simulink model "animation"  (R2018b)
settings: Solver=VariableStepAuto  StartTime=0.0  StopTime=281.0754  FixedStep=0.01  RelTol=1e-3  EnableMultiTasking=on
values from neighbouring files (symbols this model uses):
  cm = [[0.3;49.6;82],[355.2;24;0.7],[9.8;0;36.7],[0.1;246;20],[0;13.9;55],[0;0;59]]    [dynamics.m]    (also in invDynController.m)
  D = generalizedInertiaMatrix(q,rho,DH,m,cm,I)    [dynamics.m]    (also in generalizedInertiaMatrix.m = D + (Si*J(:,:,i))'*Mc_i*(Si*J(:,:,i)); invDynController.m; motionPlanning.m = size(q_new,2); trajGen.m = size(q,1))
  m = [9 4.3 1.9 1.7 0.3 0.1]    [dynamics.m]    (also in invDynController.m)
  N = numel(pos_list)    [missionPlanning.m]    (also in motionPlanning.m = size(q_new,1); simManipulator.m = numel(Path(:,1)); trajGen.m = size(q,2); trajGen_fmincon.m = size(q,2))
undefined symbols (not defined in the file or in its folder): X, Y, Z
libraries: sm_lib x142, nesl_utility x51, simulink x2
(part 1 of 4)
settings Model: Creator=USER  LastModifiedBy=rabay
settings OptimizationCC: LifeSpan=inf
settings SFSimCC: SimUseLocalCustomCode=off
settings RTWCC: RTWUseLocalCustomCode=off
settings CodeAppCC: StateflowObjectComments=on
settings SimscapeCC: SimscapeNormalizeSystem=off

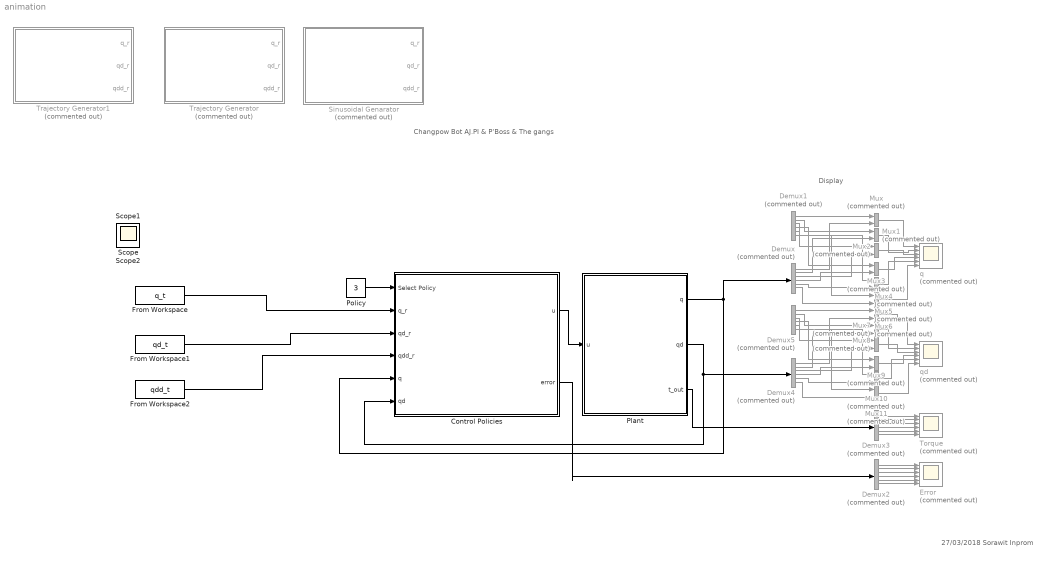
== system animation ==
  note: Display
  note: 27/03/2018
      | Sorawit Inprom
  note: Changpow Bot
      | AJ.PI & P'Boss & The gangs
  Control Policies : Subsystem  mask{Kp1=diag([10 10 10 10 10 10]), Kd1=diag([10 10 10 10 10 10]), Kp2=diag([10 10 10 10 10 10]), Kd2=diag([10 10 10 10 10 10]), max1=50, max2=30, max3=20, max4=20, max5=20, max6=20}
      mask prompts: Kp1 "Propotional Gain1"; Kd1 "Derivative Gain1"; Kp2 "Propotional Gain2"; Kd2 "Derivative Gain2"; max1 "Maximum Torque Joint1"; max2 "Maximum Torque Joint2"; max3 "Maximum Torque Joint3"; max4 "Maximum Torque Joint4"; max5 "Maximum Torque Joint5"; max6 "Maximum Torque Joint6"
      mask Display: image('C:\Users\dell\Downloads\29693766_2047918065235944_898913540_o.jpg');
  Demux{,1..5} (6 alike) : Demux  Commented=on  Outputs=6
  Error : Scope  Commented=on  NumInputPorts=6
  From Workspace : FromWorkspace  VariableName=q_t  SampleTime=0  Interpolate=off  OutputAfterFinalValue=Holding final value
  From Workspace1 : FromWorkspace  VariableName=qd_t  SampleTime=0  Interpolate=off  OutputAfterFinalValue=Holding final value
  From Workspace2 : FromWorkspace  VariableName=qdd_t  SampleTime=0  Interpolate=off  OutputAfterFinalValue=Holding final value
  Mux{,1..11} (12 alike) : Mux  Commented=on  Inputs=2
  Plant : Subsystem
  Policy : Constant  Value=3
  Sinusoidal Genarator : Subsystem  Commented=on  mask{a1=1, w1=pi*0.5}
      mask prompts: a1 "alpha"; w1 "omega"
  Torque : Scope  Commented=on  NumInputPorts=6
  Trajectory Generator : Subsystem  Commented=on  mask{T=10, q1=[2.504;0.367;0.569;-1.721;-0.122;1.7577], q2=[1.9908;-0.176;1.061;2;0.151;1.1145]}
      mask prompts: T "Time travel"; q1 "Goal Configuration Space1"; q2 "Goal Configuration Space2"
  Trajectory Generator1 : Subsystem  Commented=on  mask{T=5, q1=1, q2=0.5, q3=0.2, q4=0, q5=0, q6=0}
      mask prompts: T "Time travel"; q1 "Goal1"; q2 "Goal2"; q3 "Goal3"; q4 "Goal4"; q5 "Goal5"; q6 "Goal6"
  q : Scope  Commented=on  NumInputPorts=6
  qd : Scope  Commented=on  NumInputPorts=6
  Scope : Scope
  Scope1 : Scope
  Scope2 : Scope
  wires:
  Control Policies/1(u) -> Plant/1(u)
  Policy/1 -> Control Policies/1(Select Policy)
  Demux2/1 -> Error/1
  Demux1/5 -> Mux4/1
  Demux1/4 -> Mux3/1
  Demux3/1 -> Torque/1
  Demux3/2 -> Torque/2
  Demux3/3 -> Torque/3
  Demux/4 -> Mux3/2
  Demux/6 -> Mux5/2
  Demux1/3 -> Mux2/1
  Demux/3 -> Mux2/2
  Demux1/6 -> Mux5/1
  Demux1/2 -> Mux1/1
  Demux/1 -> Mux/2
  Control Policies/2(error) -> Demux2/1
  Demux/2 -> Mux1/2
  Mux2/1 -> q/3
  Demux/5 -> Mux4/2
  Demux5/1 -> Mux6/1
  Demux4/1 -> Mux6/2
  Mux6/1 -> qd/1
  Demux4/2 -> Mux7/2
  Demux4/3 -> Mux8/2
  Mux11/1 -> qd/6
  Mux8/1 -> qd/3
  Demux5/2 -> Mux7/1
  Mux7/1 -> qd/2
  Demux5/3 -> Mux8/1
  Mux9/1 -> qd/4
  Demux5/4 -> Mux9/1
  Demux4/4 -> Mux9/2
  Demux4/5 -> Mux10/2
  Demux5/6 -> Mux11/1
  Demux4/6 -> Mux11/2
  Demux5/5 -> Mux10/1
  Demux2/3 -> Error/3
  Demux1/1 -> Mux/1
  Demux2/2 -> Error/2
  Plant/1(q) -> Demux/1, Control Policies/5(q)
  Mux/1 -> q/1
  Plant/3(t_out) -> Demux3/1
  Mux1/1 -> q/2
  Plant/2(qd) -> Control Policies/6(qd), Demux4/1
  Mux3/1 -> q/4
  Mux4/1 -> q/5
  Mux5/1 -> q/6
  Mux10/1 -> qd/5
  Demux2/4 -> Error/4
  Demux2/5 -> Error/5
  Demux2/6 -> Error/6
  Demux3/4 -> Torque/4
  Demux3/5 -> Torque/5
  Demux3/6 -> Torque/6
  From Workspace/1 -> Control Policies/2(q_r)
  From Workspace1/1 -> Control Policies/3(qd_r)
  From Workspace2/1 -> Control Policies/4(qdd_r)

== system animation/Control Policies ==
  Select Policy : Inport
  q_r : Inport  Port=2
  qd_r : Inport  Port=3
  qdd_r : Inport  Port=4
  q : Inport  Port=5
  qd : Inport  Port=6
  Inverse Dynamics Control : Subsystem
  Mechanical Saturation : Subsystem
  Multiport Switch : MultiPortSwitch  DiagnosticForDefault=None
  PD Control : Subsystem
  PD Control with Gravity Compensator : Subsystem
  Sum : Sum  Inputs=|+-
  u : Outport
  error : Outport  Port=2
  wires:
  qd_r/1 -> PD Control/2(qd_r), Inverse Dynamics Control/2(qd_r), PD Control with Gravity Compensator/2(qd_r)
  q_r/1 -> PD Control/1(q_r), Sum/1, Inverse Dynamics Control/1(q_r), PD Control with Gravity Compensator/1(q_r)
  qdd_r/1 -> PD Control/3(qdd_r), Inverse Dynamics Control/3(qdd_r), PD Control with Gravity Compensator/3(qdd_r)
  q/1 -> PD Control/4(q), Sum/2, Inverse Dynamics Control/4(q), PD Control with Gravity Compensator/4("q ")
  qd/1 -> PD Control/5(qd), Inverse Dynamics Control/5(qd), PD Control with Gravity Compensator/5(qd)
  Select Policy/1 -> Multiport Switch/1
  Multiport Switch/1 -> Mechanical Saturation/1(t)
  Mechanical Saturation/1(t_sat) -> u/1
  Sum/1 -> error/1
  PD Control/1(u) -> Multiport Switch/2
  PD Control with Gravity Compensator/1(u) -> Multiport Switch/3
  Inverse Dynamics Control/1(u) -> Multiport Switch/4

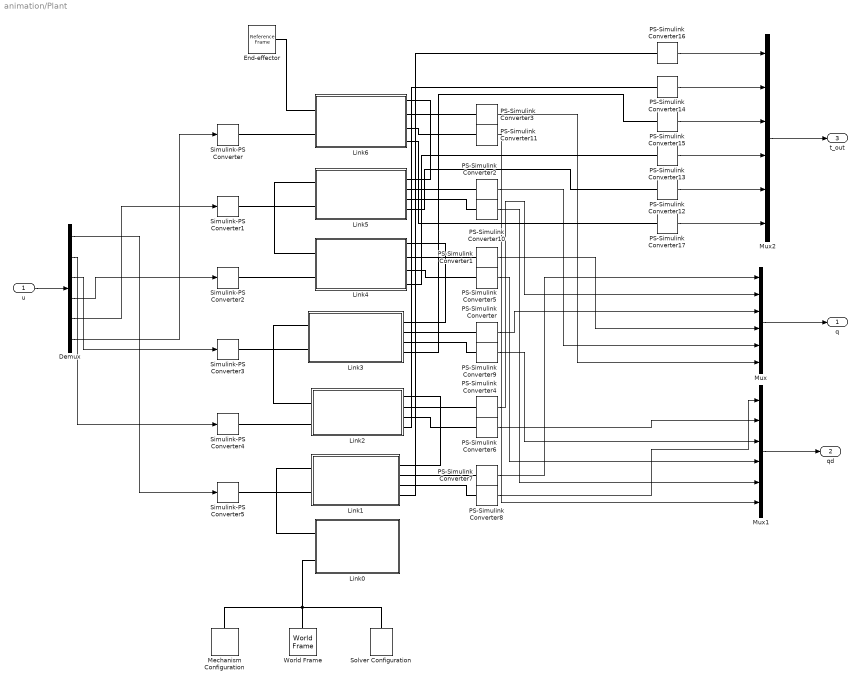
== system animation/Plant ==
  u : Inport
  Demux : Demux  Outputs=6
  End-effector : sm_lib/Frames and Transforms/Reference Frame
  Link0 : Subsystem
  Link1 : Subsystem
  Link2 : Subsystem
  Link3 : Subsystem
  Link4 : Subsystem
  Link5 : Subsystem
  Link6 : Subsystem
  Mechanism Configuration : sm_lib/Utilities/Mechanism Configuration  UniformGravity=Constant  GravityVector=[0 0 -9.80665]  GravityUnits=m/s^2  LinearizationDelta=0.001
  Mux : Mux  Inputs=6
  Mux1 : Mux  Inputs=6
  Mux2 : Mux  Inputs=6
  PS-Simulink Converter{,1..17} (18 alike) : nesl_utility/PS-Simulink Converter  PhysicalDomain=network_engine_domain  SubClassName=ps_output  LeftPortType=input  RightPortType=output  PseudoPeriodic=off  Frequencies=[]  Unit=1  AffineConversion=off
  Simulink-PS Converter{,1..5} (6 alike) : nesl_utility/Simulink-PS Converter  PhysicalDomain=network_engine_domain  SubClassName=ps_input  LeftPortType=input  RightPortType=output  PseudoPeriodic=off  Frequencies=[]  NoiseDistribution=none  NoiseParameters=[]  Unit=1  AffineConversion=off  FilteringAndDerivatives=zero  SimscapeFilterOrder=1  InputFilterTimeConstant=0.001  UdotUserProvided=1
  Solver Configuration : nesl_utility/Solver Configuration  PhysicalDomain=network_engine_domain  SubClassName=solver  LeftPortType=input  RightPortType=generic  Tones=[]  Harmonics=[]  SimulateNoise=off  Profile=off  UseLocalSampling=off  EnableSwitchedLinearOptims=on  FrequencyDomain=off  UseCCode=off  RelTol=0.001  AbsTol=1e-06  MinStep=1e-09  ToWorkspace=off  RevertToSquareIcSolve=off  NumHomotopyIterations=100  PhasorMode=off  PhasorModeNumHarmonics=1  DoDC=off  ResidualTolerance=1e-09  UseLocalSolver=off  LocalSolverChoice=NE_BACKWARD_EULER_ADVANCER  LocalSolverSampleTime=0.001  DoFixedCost=off  MaxNonlinIter=3  MaxModeIter=2  LinearAlgebra=Sparse  EquationFormulation=NE_TIME_EF  DelaysMemoryBudget=1024  AutomaticFiltering=on  FilteringTimeConstant=0.001  PartitionStorageMethod=AS_NEEDED  PartitionMemoryBudget=1024
  World Frame : sm_lib/Frames and Transforms/World Frame
  q : Outport
  qd : Outport  Port=2
  t_out : Outport  Port=3
  wires:
  Mux/1 -> q/1
  u/1 -> Demux/1
  Mux1/1 -> qd/1
  Mux2/1 -> t_out/1
  PS-Simulink Converter17/1 -> Mux2/6
  PS-Simulink Converter14/1 -> Mux2/2
  PS-Simulink Converter16/1 -> Mux2/1
  PS-Simulink Converter15/1 -> Mux2/3
  PS-Simulink Converter13/1 -> Mux2/4
  PS-Simulink Converter12/1 -> Mux2/5
  Demux/1 -> Simulink-PS Converter5/1
  Demux/2 -> Simulink-PS Converter4/1
  Demux/3 -> Simulink-PS Converter3/1
  Demux/4 -> Simulink-PS Converter2/1
  Demux/5 -> Simulink-PS Converter1/1
  Demux/6 -> Simulink-PS Converter/1
  PS-Simulink Converter3/1 -> Mux/6
  PS-Simulink Converter2/1 -> Mux/5
  PS-Simulink Converter1/1 -> Mux/4
  PS-Simulink Converter/1 -> Mux/3
  PS-Simulink Converter4/1 -> Mux/2
  PS-Simulink Converter7/1 -> Mux/1
  PS-Simulink Converter11/1 -> Mux1/6
  PS-Simulink Converter8/1 -> Mux1/1
  PS-Simulink Converter6/1 -> Mux1/2
  PS-Simulink Converter9/1 -> Mux1/3
  PS-Simulink Converter5/1 -> Mux1/4
  PS-Simulink Converter10/1 -> Mux1/5
  connections:
  World Frame/RConn1 -- Solver Configuration/RConn1 -- Link0/LConn2 -- Mechanism Configuration/RConn1
  Link1/RConn2 -- PS-Simulink Converter7/LConn1
  Link6/RConn2 -- PS-Simulink Converter3/LConn1
  Link3/RConn2 -- PS-Simulink Converter/LConn1
  Link2/RConn2 -- PS-Simulink Converter4/LConn1
  Simulink-PS Converter5/RConn1 -- Link1/LConn2
  Simulink-PS Converter4/RConn1 -- Link2/LConn2
  Link2/RConn1 -- Link1/RConn1
  Link1/LConn1 -- Link0/LConn1
  Simulink-PS Converter/RConn1 -- Link6/LConn2
  Simulink-PS Converter3/RConn1 -- Link3/LConn2
  Simulink-PS Converter2/RConn1 -- Link4/LConn2
  Simulink-PS Converter1/RConn1 -- Link5/LConn2
  Link4/RConn3 -- PS-Simulink Converter5/LConn1
  Link6/RConn3 -- PS-Simulink Converter11/LConn1
  Link5/RConn2 -- PS-Simulink Converter2/LConn1
  PS-Simulink Converter10/LConn1 -- Link5/RConn3
  PS-Simulink Converter8/LConn1 -- Link1/RConn3
  Link4/RConn1 -- Link3/RConn1
  Link5/LConn1 -- Link4/LConn1
  Link6/RConn1 -- Link5/RConn1
  Link3/LConn1 -- Link2/LConn1
  Link4/RConn2 -- PS-Simulink Converter1/LConn1
  PS-Simulink Converter9/LConn1 -- Link3/RConn3
  PS-Simulink Converter6/LConn1 -- Link2/RConn3
  End-effector/RConn1 -- Link6/LConn1
  Link6/RConn4 -- PS-Simulink Converter17/LConn1
  Link5/RConn4 -- PS-Simulink Converter12/LConn1
  Link4/RConn4 -- PS-Simulink Converter13/LConn1
  Link3/RConn4 -- PS-Simulink Converter15/LConn1
  Link2/RConn4 -- PS-Simulink Converter14/LConn1
  Link1/RConn4 -- PS-Simulink Converter16/LConn1

== system animation/Sinusoidal Genarator ==
  Clock : Clock
  Mux : Mux  Inputs=6
  Mux1 : Mux  Inputs=6
  Mux2 : Mux  Inputs=6
  Sin : Trigonometry
  Sin1 : Trigonometry  Operator=cos
  a1 : Gain  Gain=a1
  w1 : Gain  Gain=w1
  w3 : Gain  Gain=a1*w1
  w6 : Gain  Gain=-a1*w1^2
  q_r : Outport
  qd_r : Outport  Port=2
  qdd_r : Outport  Port=3
  wires:
  w3/1 -> Mux1/6, Mux1/5, Mux1/4, Mux1/3, Mux1/2, Mux1/1  "a1w1cos(w1t)"
  Sin/1 -> w6/1, a1/1
  w1/1 -> Sin1/1, Sin/1
  Clock/1 -> w1/1
  Mux/1 -> q_r/1
  Sin1/1 -> w3/1
  Mux1/1 -> qd_r/1
  Mux2/1 -> qdd_r/1
  w6/1 -> Mux2/6, Mux2/5, Mux2/4, Mux2/3, Mux2/2, Mux2/1  "-a1w1^2sin(w1t)"
  a1/1 -> Mux/6, Mux/5, Mux/4, Mux/3, Mux/2, Mux/1  "a1sin(w1t)"

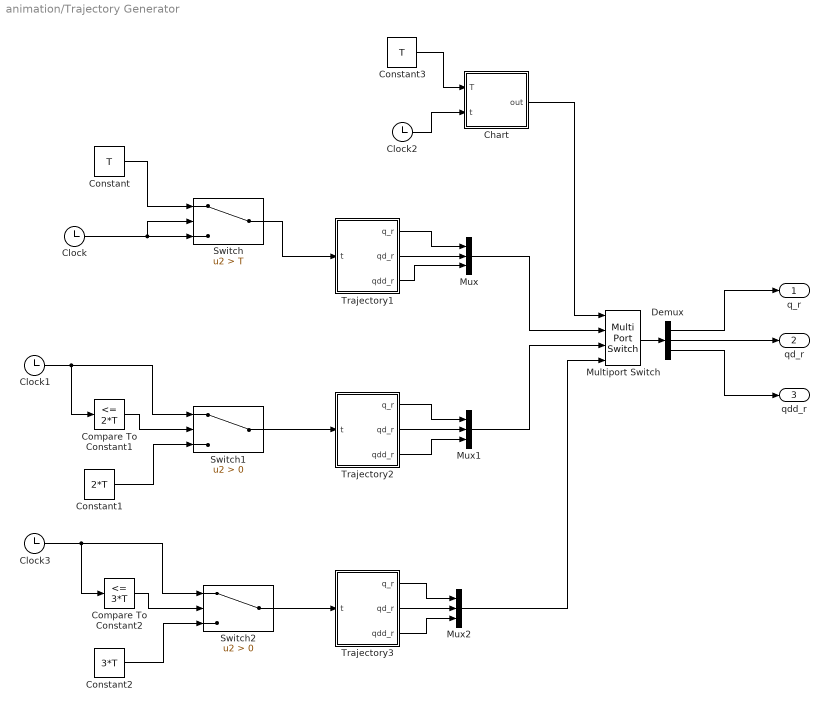
== system animation/Trajectory Generator ==
  Chart : Stateflow chart  TreatAsAtomicUnit=on
  Clock{,1..3} (4 alike) : Clock
  Compare To Constant1 : simulink/Logic and Bit Operations/Compare To Constant  relop=<=  const=2*T  OutDataTypeStr=uint8
  Compare To Constant2 : simulink/Logic and Bit Operations/Compare To Constant  relop=<=  const=3*T  OutDataTypeStr=uint8
  Constant : Constant  Value=T
  Constant1 : Constant  Value=2*T
  Constant2 : Constant  Value=3*T
  Constant3 : Constant  Value=T
  Demux : Demux  Outputs=3
  Multiport Switch : MultiPortSwitch  DiagnosticForDefault=None
  Mux : Mux  Inputs=3
  Mux1 : Mux  Inputs=3
  Mux2 : Mux  Inputs=3
  Switch : Switch  Criteria=u2 > Threshold  Threshold=T
  Switch1 : Switch  Criteria=u2 > Threshold
  Switch2 : Switch  Criteria=u2 > Threshold
  Trajectory1 : Subsystem
  Trajectory2 : Subsystem
  Trajectory3 : Subsystem
  q_r : Outport
  qd_r : Outport  Port=2
  qdd_r : Outport  Port=3
  wires:
  Clock/1 -> Switch/2, Switch/3
  Constant/1 -> Switch/1
  Switch/1 -> Trajectory1/1(t)
  Switch1/1 -> Trajectory2/1(t)
  Trajectory1/1(q_r) -> Mux/1
  Trajectory1/2(qd_r) -> Mux/2
  Trajectory1/3(qdd_r) -> Mux/3
  Trajectory2/2(qd_r) -> Mux1/2
  Trajectory2/1(q_r) -> Mux1/1
  Trajectory2/3(qdd_r) -> Mux1/3
  Mux/1 -> Multiport Switch/2
  Mux1/1 -> Multiport Switch/3
  Clock2/1 -> Chart/2(t)
  Multiport Switch/1 -> Demux/1
  Constant1/1 -> Switch1/3
  Clock1/1 -> Switch1/1, Compare To Constant1/1
  Compare To Constant1/1 -> Switch1/2
  Compare To Constant2/1 -> Switch2/2
  Clock3/1 -> Compare To Constant2/1, Switch2/1
  Constant2/1 -> Switch2/3
  Switch2/1 -> Trajectory3/1(t)
  Trajectory3/2(qd_r) -> Mux2/2
  Trajectory3/1(q_r) -> Mux2/1
  Trajectory3/3(qdd_r) -> Mux2/3
  Mux2/1 -> Multiport Switch/4
  Constant3/1 -> Chart/1(T)
  Chart/1(out) -> Multiport Switch/1
  Demux/1 -> q_r/1
  Demux/2 -> qd_r/1
  Demux/3 -> qdd_r/1

== system animation/Trajectory Generator1 ==
  Clock1 : Clock
  Constant1 : Constant  Value=T
  Switch1 : Switch  Criteria=u2 > Threshold  Threshold=T
  Trajectory2 : Subsystem
  q_r : Outport
  qd_r : Outport  Port=2
  qdd_r : Outport  Port=3
  wires:
  Trajectory2/3(qdd_r) -> qdd_r/1
  Constant1/1 -> Switch1/1
  Trajectory2/1(q_r) -> q_r/1
  Clock1/1 -> Switch1/2, Switch1/3
  Trajectory2/2(qd_r) -> qd_r/1
  Switch1/1 -> Trajectory2/1(t)

== system animation/Control Policies/Inverse Dynamics Control ==
  q_r : Inport
  qd_r : Inport  Port=2
  qdd_r : Inport  Port=3
  q : Inport  Port=4
  qd : Inport  Port=5
  Inverse Dynamics : Subsystem
  Outer_loop : Subsystem
  u : Outport
  wires:
  qd_r/1 -> Outer_loop/2(qd_r)
  q/1 -> Inverse Dynamics/2(q), Outer_loop/4(q)
  qd/1 -> Inverse Dynamics/3(qd), Outer_loop/5(qd)
  Outer_loop/1(a) -> Inverse Dynamics/1(a)
  qdd_r/1 -> Outer_loop/3(qdd_r)
  q_r/1 -> Outer_loop/1(q_r)
  Inverse Dynamics/1("Torque ") -> u/1

== system animation/Control Policies/Mechanical Saturation ==
  t : Inport
  Demux3 : Demux  Outputs=6
  Mux : Mux  Inputs=6
  Saturation : Saturate  UpperLimit=max1  LowerLimit=-max1
  Saturation1 : Saturate  UpperLimit=max2  LowerLimit=-max2
  Saturation2 : Saturate  UpperLimit=max3  LowerLimit=-max3
  Saturation3 : Saturate  UpperLimit=max4  LowerLimit=-max4
  Saturation4 : Saturate  UpperLimit=max5  LowerLimit=-max5
  Saturation5 : Saturate  UpperLimit=max6  LowerLimit=-max6
  t_sat : Outport
  wires:
  Demux3/3 -> Saturation2/1
  Saturation2/1 -> Mux/3
  t/1 -> Demux3/1
  Demux3/4 -> Saturation3/1
  Saturation3/1 -> Mux/4
  Demux3/2 -> Saturation1/1
  Saturation/1 -> Mux/1
  Saturation1/1 -> Mux/2
  Demux3/6 -> Saturation5/1
  Saturation5/1 -> Mux/6
  Demux3/5 -> Saturation4/1
  Mux/1 -> t_sat/1
  Saturation4/1 -> Mux/5
  Demux3/1 -> Saturation/1

== system animation/Control Policies/PD Control ==
  q_r : Inport
  qd_r : Inport  Port=2
  qdd_r : Inport  Port=3
  q : Inport  Port=4
  qd : Inport  Port=5
  Kd3 : Gain  Gain=Kd2  Multiplication=Matrix(K*u)
  Kp3 : Gain  Gain=Kp2  Multiplication=Matrix(K*u)
  Sum12 : Sum  Inputs=|+-
  Sum13 : Sum  Inputs=|++
  Sum8 : Sum  Inputs=|+-
  u : Outport
  wires:
  q_r/1 -> Sum8/1
  qd/1 -> Sum12/2
  Kd3/1 -> Sum13/2
  qd_r/1 -> Sum12/1
  Sum12/1 -> Kd3/1  "eqd"
  q/1 -> Sum8/2
  Kp3/1 -> Sum13/1
  Sum8/1 -> Kp3/1  "eq"
  Sum13/1 -> u/1

== system animation/Control Policies/PD Control with Gravity Compensator ==
  q_r : Inport
  qd_r : Inport  Port=2
  qdd_r : Inport  Port=3
  "q " : Inport  Port=4
  qd : Inport  Port=5
  Gravity Compensator : Subsystem
  PD control : Subsystem
  u : Outport
  wires:
  PD control/1(u) -> u/1
  Gravity Compensator/1("Torque ") -> PD control/1(compensate)
  q_r/1 -> PD control/2(q_r)
  qd/1 -> PD control/5(qd)
  qd_r/1 -> PD control/3(qd_r)
  "q "/1 -> PD control/4(q), Gravity Compensator/1(q)

== system animation/Plant/Link0 ==
  Rigid Transform : sm_lib/Frames and Transforms/Rigid Transform  TranslationMethod=None  TranslationStandardOffset=0  TranslationLengthUnit=m  TranslationStandardAxis=+Z  TranslationCartesianOffset=[0 0 0]  TranslationROffset=0  TranslationROffsetUnits=m  TranslationZOffset=0  TranslationZOffsetUnits=m  TranslationThetaOffset=0  TranslationThetaOffsetUnits=deg  RotationMethod=StandardAxis  RotationAngleUnits=rad  RotationStandardAxis=+Z  RotationAngle=pi  RotationArbitraryAxis=[0 0 1]  FollAlignAxisA=+X  BaseAlignAxisA=+Y  FollAlignAxisB=+Y  BaseAlignAxisB=+Z  RotationSequenceAxes=FollowerAxes  RotationSequence=XYX  RotationSequenceAngles=[0 0 0]  RotationSequenceAnglesUnits=deg  RotationMatrix=[1 0 0; 0 1 0; 0 0 1]
  Solid : sm_lib/Body Elements/Solid  InertiaType=Custom  Mass=12.21  MassUnits=kg  CenterOfMass=[53.3 2.09 37.75]  CenterOfMassUnits=mm  MomentsOfInertia=[0.27 0.33 0.54]  MomentsOfInertiaUnits=kg*m^2  ProductsOfInertia=[0 0.03 0.01]  ProductsOfInertiaUnits=kg*m^2  BasedOnType=Density  Density=1000  DensityUnits=kg/m^3  DoExposeReferenceFrame=on  SerializedFrames=<Frames/>  GraphicType=FromGeometry  MarkerShape=Sphere  MarkerSize=10  GraphicVisPropType=SimpleVisualProperties  GraphicDiffuseColor=[0.5 0.5 0.5]  GraphicSpecularColor=[0.5 0.5 0.5 1.0]  GraphicAmbientColor=[0.15 0.15 0.15 1.0]  GraphicEmissiveColor=[0.0 0.0 0.0 1.0]  GraphicShininess=75  GraphicOpacity=1.0  GeometryShape=FromFile  RectangleSize=[1 1]  RectangleSizeUnits=m  BrickDimensions=[1 1 1]  BrickDimensionUnits=m  CylinderRadius=1  CylinderRadiusUnits=m  CylinderLength=1  CylinderLengthUnits=m  SphereRadius=1  SphereRadiusUnits=m  EllipsoidRadii=[1 1 1]  EllipsoidRadiiUnits=m  ExtrusionCrossSection=[1 1; -1 1; -1 -1; 1 -1]  ExtrusionCrossSectionUnits=m  ExtrusionLength=1  ExtrusionLengthUnits=m  PolygonNumSides=3  PolygonOuterRadius=1  PolygonOuterRadiusUnits=m  ExtGeomFileType=STL  ExtGeomFileName=C:\Users\dell\Desktop\module8&9\Intro to robotics\Project\CAD\Assem0+frame.STL  ExtGeomFileUnits=mm  RevolutionCrossSection=[1 1; 1 -1; 2 -1; 2 1]  RevolutionCrossSectionUnits=m  RevolutionExtent=Full  RevolutionAngle=180  RevolutionAngleUnits=deg
  Solid1 : sm_lib/Body Elements/Solid  InertiaType=Custom  Mass=1  MassUnits=kg  CenterOfMass=[0 0 0]  CenterOfMassUnits=m  MomentsOfInertia=[1 1 1]  MomentsOfInertiaUnits=kg*m^2  ProductsOfInertia=[0 0 0]  ProductsOfInertiaUnits=kg*m^2  BasedOnType=Density  Density=1000  DensityUnits=kg/(m^3)  DoExposeReferenceFrame=on  SerializedFrames=<Frames/>  GraphicType=FromGeometry  MarkerShape=Sphere  MarkerSize=10  GraphicVisPropType=SimpleVisualProperties  GraphicDiffuseColor=[0.5 0.5 0.5]  GraphicSpecularColor=[0.5 0.5 0.5 1.0]  GraphicAmbientColor=[0.15 0.15 0.15 1.0]  GraphicEmissiveColor=[0.0 0.0 0.0 1.0]  GraphicShininess=75  GraphicOpacity=1.0  GeometryShape=FromFile  RectangleSize=[1 1]  RectangleSizeUnits=m  BrickDimensions=[1 1 1]  BrickDimensionUnits=m  CylinderRadius=1  CylinderRadiusUnits=m  CylinderLength=1  CylinderLengthUnits=m  SphereRadius=1  SphereRadiusUnits=m  EllipsoidRadii=[1 1 1]  EllipsoidRadiiUnits=m  ExtrusionCrossSection=[1 1; -1 1; -1 -1; 1 -1]  ExtrusionCrossSectionUnits=m  ExtrusionLength=1  ExtrusionLengthUnits=m  PolygonNumSides=3  PolygonOuterRadius=1  PolygonOuterRadiusUnits=m  ExtGeomFileType=STL  ExtGeomFileName=D:\Chin\3rdYearsProject\IntroRobotics\Project\CAD\Workspace_with_Plate.STL  ExtGeomFileUnits=mm  RevolutionCrossSection=[1 1; 1 -1; 2 -1; 2 1]  RevolutionCrossSectionUnits=m  RevolutionExtent=Full  RevolutionAngle=180  RevolutionAngleUnits=deg
  Frame0 : PMIOPort  Side=Left
  World Frame : PMIOPort  Port=2  Side=Left
  connections:
  Solid/RConn1 -- Solid1/RConn1 -- Rigid Transform/RConn1 -- Frame0/RConn1
  World Frame/RConn1 -- Rigid Transform/LConn1

== system animation/Plant/Link1 ==
  Reference Frame : sm_lib/Frames and Transforms/Reference Frame
  Revolute Joint : sm_lib/Joints/Revolute Joint  SenseConstraintForce=off  SenseConstraintForceX=off  SenseConstraintForceY=off  SenseConstraintForceZ=off  SenseConstraintTorque=off  SenseConstraintTorqueX=off  SenseConstraintTorqueY=off  SenseConstraintTorqueZ=off  SenseTotalForce=off  SenseTotalForceX=off  SenseTotalForceY=off  SenseTotalForceZ=off  SenseTotalTorque=off  SenseTotalTorqueX=off  SenseTotalTorqueY=off  SenseTotalTorqueZ=off  CompositeWrenchDir=FollowerOnBase  CompositeWrenchFrame=BaseFrame  EquilibriumPosition=0  EquilibriumPositionUnits=deg  SpringStiffness=0  SpringStiffnessUnits=N*m/deg  DampingCoefficient=0  DampingCoefficientUnits=N*m/(deg/s)  TorqueActuationMode=InputTorque  MotionActuationMode=ComputedMotion  SensePosition=on  SenseVelocity=on  SenseAcceleration=off  SenseTorqueForce=on  PositionTargetSpecify=on  PositionTargetPriority=High  PositionTargetValue=0  PositionTargetValueUnits=deg  VelocityTargetSpecify=on  VelocityTargetPriority=High  VelocityTargetValue=0  VelocityTargetValueUnits=deg/s
  Rigid Transform1 : sm_lib/Frames and Transforms/Rigid Transform  TranslationMethod=None  TranslationStandardOffset=0  TranslationLengthUnit=m  TranslationStandardAxis=+Z  TranslationCartesianOffset=[0 0 0]  TranslationROffset=0  TranslationROffsetUnits=m  TranslationZOffset=0  TranslationZOffsetUnits=m  TranslationThetaOffset=0  TranslationThetaOffsetUnits=deg  RotationMethod=StandardAxis  RotationAngleUnits=rad  RotationStandardAxis=+Z  RotationAngle=-pi/2  RotationArbitraryAxis=[0 0 1]  FollAlignAxisA=+X  BaseAlignAxisA=+Y  FollAlignAxisB=+Y  BaseAlignAxisB=+Z  RotationSequenceAxes=FollowerAxes  RotationSequence=XYX  RotationSequenceAngles=[0 0 0]  RotationSequenceAnglesUnits=deg  RotationMatrix=[1 0 0; 0 1 0; 0 0 1]
  Rigid Transform17 : sm_lib/Frames and Transforms/Rigid Transform  TranslationMethod=None  TranslationStandardOffset=500  TranslationLengthUnit=mm  TranslationStandardAxis=+X  TranslationCartesianOffset=[0 0 0]  TranslationROffset=0  TranslationROffsetUnits=m  TranslationZOffset=0  TranslationZOffsetUnits=m  TranslationThetaOffset=0  TranslationThetaOffsetUnits=deg  RotationMethod=StandardAxis  RotationAngleUnits=rad  RotationStandardAxis=+X  RotationAngle=pi/2  RotationArbitraryAxis=[0 0 1]  FollAlignAxisA=+X  BaseAlignAxisA=+Y  FollAlignAxisB=+Y  BaseAlignAxisB=+Z  RotationSequenceAxes=FollowerAxes  RotationSequence=XYX  RotationSequenceAngles=[0 0 0]  RotationSequenceAnglesUnits=deg  RotationMatrix=[1 0 0; 0 1 0; 0 0 1]
  Rigid Transform2 : sm_lib/Frames and Transforms/Rigid Transform  TranslationMethod=StandardAxis  TranslationStandardOffset=250.5  TranslationLengthUnit=mm  TranslationStandardAxis=+Z  TranslationCartesianOffset=[0 0 0]  TranslationROffset=0  TranslationROffsetUnits=m  TranslationZOffset=0  TranslationZOffsetUnits=m  TranslationThetaOffset=0  TranslationThetaOffsetUnits=deg  RotationMethod=None  RotationAngleUnits=deg  RotationStandardAxis=+Z  RotationAngle=0.0  RotationArbitraryAxis=[0 0 1]  FollAlignAxisA=+X  BaseAlignAxisA=+Y  FollAlignAxisB=+Y  BaseAlignAxisB=+Z  RotationSequenceAxes=FollowerAxes  RotationSequence=XYX  RotationSequenceAngles=[0 0 0]  RotationSequenceAnglesUnits=deg  RotationMatrix=[1 0 0; 0 1 0; 0 0 1]
  Rigid Transform3 : sm_lib/Frames and Transforms/Rigid Transform  TranslationMethod=None  TranslationStandardOffset=0  TranslationLengthUnit=m  TranslationStandardAxis=+Z  TranslationCartesianOffset=[0 0 0]  TranslationROffset=0  TranslationROffsetUnits=m  TranslationZOffset=0  TranslationZOffsetUnits=m  TranslationThetaOffset=0  TranslationThetaOffsetUnits=deg  RotationMethod=None  RotationAngleUnits=rad  RotationStandardAxis=+X  RotationAngle=pi/2  RotationArbitraryAxis=[0 0 1]  FollAlignAxisA=+X  BaseAlignAxisA=+Y  FollAlignAxisB=+Y  BaseAlignAxisB=+Z  RotationSequenceAxes=FollowerAxes  RotationSequence=XYX  RotationSequenceAngles=[0 0 0]  RotationSequenceAnglesUnits=deg  RotationMatrix=[1 0 0; 0 1 0; 0 0 1]
  Solid1 : sm_lib/Body Elements/Solid  InertiaType=Custom  Mass=8.44  MassUnits=kg  CenterOfMass=[0.26 -62.55 100.99]  CenterOfMassUnits=mm  MomentsOfInertia=[0.25 0.21 0.09]  MomentsOfInertiaUnits=kg*m^2  ProductsOfInertia=[-0.02 0 0]  ProductsOfInertiaUnits=kg*m^2  BasedOnType=Density  Density=1000  DensityUnits=kg/m^3  DoExposeReferenceFrame=on  SerializedFrames=<Frames/>  GraphicType=FromGeometry  MarkerShape=Sphere  MarkerSize=10  GraphicVisPropType=SimpleVisualProperties  GraphicDiffuseColor=[0.0 0.0 1.0]  GraphicSpecularColor=[0.5 0.5 0.5 1.0]  GraphicAmbientColor=[0.15 0.15 0.15 1.0]  GraphicEmissiveColor=[0.0 0.0 0.0 1.0]  GraphicShininess=75  GraphicOpacity=1.0  GeometryShape=FromFile  RectangleSize=[1 1]  RectangleSizeUnits=m  BrickDimensions=[1 1 1]  BrickDimensionUnits=m  CylinderRadius=1  CylinderRadiusUnits=m  CylinderLength=1  CylinderLengthUnits=m  SphereRadius=1  SphereRadiusUnits=m  EllipsoidRadii=[1 1 1]  EllipsoidRadiiUnits=m  ExtrusionCrossSection=[1 1; -1 1; -1 -1; 1 -1]  ExtrusionCrossSectionUnits=m  ExtrusionLength=1  ExtrusionLengthUnits=m  PolygonNumSides=3  PolygonOuterRadius=1  PolygonOuterRadiusUnits=m  ExtGeomFileType=STL  ExtGeomFileName=D:\Chin\3rdYearsProject\IntroRobotics\Project\CAD\Assem2+1.STL  ExtGeomFileUnits=mm  RevolutionCrossSection=[1 1; 1 -1; 2 -1; 2 1]  RevolutionCrossSectionUnits=m  RevolutionExtent=Full  RevolutionAngle=180  RevolutionAngleUnits=deg
  Frame1 : PMIOPort  Side=Right
  Frame0 : PMIOPort  Port=2  Side=Left
  q : PMIOPort  Port=3  Side=Right
  w : PMIOPort  Port=4  Side=Right
  t : PMIOPort  Port=5  Side=Left
  t_out : PMIOPort  Port=6  Side=Right
  connections:
  Rigid Transform17/RConn1 -- Frame1/RConn1 -- Solid1/RConn1 -- Reference Frame/RConn1
  Rigid Transform3/RConn1 -- Rigid Transform17/LConn1
  Rigid Transform3/LConn1 -- Rigid Transform2/RConn1
  Rigid Transform1/LConn1 -- Revolute Joint/RConn1
  Rigid Transform2/LConn1 -- Rigid Transform1/RConn1
  Revolute Joint/RConn2 -- q/RConn1
  Revolute Joint/LConn1 -- Frame0/RConn1
  Revolute Joint/RConn3 -- w/RConn1
  t/RConn1 -- Revolute Joint/LConn2
  Revolute Joint/RConn4 -- t_out/RConn1

== system animation/Plant/Link2 ==
  Reference Frame1 : sm_lib/Frames and Transforms/Reference Frame
  Revolute Joint1 : sm_lib/Joints/Revolute Joint  SenseConstraintForce=off  SenseConstraintForceX=off  SenseConstraintForceY=off  SenseConstraintForceZ=off  SenseConstraintTorque=off  SenseConstraintTorqueX=off  SenseConstraintTorqueY=off  SenseConstraintTorqueZ=off  SenseTotalForce=off  SenseTotalForceX=off  SenseTotalForceY=off  SenseTotalForceZ=off  SenseTotalTorque=off  SenseTotalTorqueX=off  SenseTotalTorqueY=off  SenseTotalTorqueZ=off  CompositeWrenchDir=FollowerOnBase  CompositeWrenchFrame=BaseFrame  EquilibriumPosition=0  EquilibriumPositionUnits=deg  SpringStiffness=0  SpringStiffnessUnits=N*m/deg  DampingCoefficient=0  DampingCoefficientUnits=N*m/(deg/s)  TorqueActuationMode=InputTorque  MotionActuationMode=ComputedMotion  SensePosition=on  SenseVelocity=on  SenseAcceleration=off  SenseTorqueForce=on  PositionTargetSpecify=on  PositionTargetPriority=High  PositionTargetValue=0  PositionTargetValueUnits=deg  VelocityTargetSpecify=on  VelocityTargetPriority=High  VelocityTargetValue=0  VelocityTargetValueUnits=deg/s
  Rigid Transform16 : sm_lib/Frames and Transforms/Rigid Transform  TranslationMethod=None  TranslationStandardOffset=500  TranslationLengthUnit=mm  TranslationStandardAxis=+X  TranslationCartesianOffset=[0 0 0]  TranslationROffset=0  TranslationROffsetUnits=m  TranslationZOffset=0  TranslationZOffsetUnits=m  TranslationThetaOffset=0  TranslationThetaOffsetUnits=deg  RotationMethod=None  RotationAngleUnits=deg  RotationStandardAxis=+Z  RotationAngle=0.0  RotationArbitraryAxis=[0 0 1]  FollAlignAxisA=+X  BaseAlignAxisA=+Y  FollAlignAxisB=+Y  BaseAlignAxisB=+Z  RotationSequenceAxes=FollowerAxes  RotationSequence=XYX  RotationSequenceAngles=[0 0 0]  RotationSequenceAnglesUnits=deg  RotationMatrix=[1 0 0; 0 1 0; 0 0 1]
  Rigid Transform4 : sm_lib/Frames and Transforms/Rigid Transform  TranslationMethod=None  TranslationStandardOffset=0  TranslationLengthUnit=m  TranslationStandardAxis=+Z  TranslationCartesianOffset=[0 0 0]  TranslationROffset=0  TranslationROffsetUnits=m  TranslationZOffset=0  TranslationZOffsetUnits=m  TranslationThetaOffset=0  TranslationThetaOffsetUnits=deg  RotationMethod=StandardAxis  RotationAngleUnits=rad  RotationStandardAxis=+Z  RotationAngle=pi/2  RotationArbitraryAxis=[0 0 1]  FollAlignAxisA=+X  BaseAlignAxisA=+Y  FollAlignAxisB=+Y  BaseAlignAxisB=+Z  RotationSequenceAxes=FollowerAxes  RotationSequence=XYX  RotationSequenceAngles=[0 0 0]  RotationSequenceAnglesUnits=deg  RotationMatrix=[1 0 0; 0 1 0; 0 0 1]
  Rigid Transform5 : sm_lib/Frames and Transforms/Rigid Transform  TranslationMethod=None  TranslationStandardOffset=500  TranslationLengthUnit=mm  TranslationStandardAxis=+X  TranslationCartesianOffset=[0 0 0]  TranslationROffset=0  TranslationROffsetUnits=m  TranslationZOffset=0  TranslationZOffsetUnits=m  TranslationThetaOffset=0  TranslationThetaOffsetUnits=deg  RotationMethod=None  RotationAngleUnits=deg  RotationStandardAxis=+Z  RotationAngle=0.0  RotationArbitraryAxis=[0 0 1]  FollAlignAxisA=+X  BaseAlignAxisA=+Y  FollAlignAxisB=+Y  BaseAlignAxisB=+Z  RotationSequenceAxes=FollowerAxes  RotationSequence=XYX  RotationSequenceAngles=[0 0 0]  RotationSequenceAnglesUnits=deg  RotationMatrix=[1 0 0; 0 1 0; 0 0 1]
  Rigid Transform6 : sm_lib/Frames and Transforms/Rigid Transform  TranslationMethod=StandardAxis  TranslationStandardOffset=500  TranslationLengthUnit=mm  TranslationStandardAxis=+X  TranslationCartesianOffset=[0 0 0]  TranslationROffset=0  TranslationROffsetUnits=m  TranslationZOffset=0  TranslationZOffsetUnits=m  TranslationThetaOffset=0  TranslationThetaOffsetUnits=deg  RotationMethod=None  RotationAngleUnits=deg  RotationStandardAxis=+Z  RotationAngle=0.0  RotationArbitraryAxis=[0 0 1]  FollAlignAxisA=+X  BaseAlignAxisA=+Y  FollAlignAxisB=+Y  BaseAlignAxisB=+Z  RotationSequenceAxes=FollowerAxes  RotationSequence=XYX  RotationSequenceAngles=[0 0 0]  RotationSequenceAnglesUnits=deg  RotationMatrix=[1 0 0; 0 1 0; 0 0 1]
  Solid2 : sm_lib/Body Elements/Solid  InertiaType=Custom  Mass=4.3  MassUnits=kg  CenterOfMass=[-355.21 24.04 0.66]  CenterOfMassUnits=mm  MomentsOfInertia=[0.02 0.64 0.65]  MomentsOfInertiaUnits=kg*m^2  ProductsOfInertia=[0 0 -0.04]  ProductsOfInertiaUnits=kg*m^2  BasedOnType=Density  Density=1000  DensityUnits=kg/m^3  DoExposeReferenceFrame=on  SerializedFrames=<Frames/>  GraphicType=FromGeometry  MarkerShape=Sphere  MarkerSize=10  GraphicVisPropType=SimpleVisualProperties  GraphicDiffuseColor=[1.0 0.0 1.0]  GraphicSpecularColor=[0.5 0.5 0.5 1.0]  GraphicAmbientColor=[0.15 0.15 0.15 1.0]  GraphicEmissiveColor=[0.0 0.0 0.0 1.0]  GraphicShininess=75  GraphicOpacity=1.0  GeometryShape=FromFile  RectangleSize=[1 1]  RectangleSizeUnits=m  BrickDimensions=[1 1 1]  BrickDimensionUnits=m  CylinderRadius=1  CylinderRadiusUnits=m  CylinderLength=1  CylinderLengthUnits=m  SphereRadius=1  SphereRadiusUnits=m  EllipsoidRadii=[1 1 1]  EllipsoidRadiiUnits=m  ExtrusionCrossSection=[1 1; -1 1; -1 -1; 1 -1]  ExtrusionCrossSectionUnits=m  ExtrusionLength=1  ExtrusionLengthUnits=m  PolygonNumSides=3  PolygonOuterRadius=1  PolygonOuterRadiusUnits=m  ExtGeomFileType=STL  ExtGeomFileName=D:\Chin\3rdYearsProject\IntroRobotics\Project\CAD\SubAssem3.STL  ExtGeomFileUnits=mm  RevolutionCrossSection=[1 1; 1 -1; 2 -1; 2 1]  RevolutionCrossSectionUnits=m  RevolutionExtent=Full  RevolutionAngle=180  RevolutionAngleUnits=deg
  Frame2 : PMIOPort  Side=Left
  Frame1 : PMIOPort  Port=2  Side=Right
  q : PMIOPort  Port=3  Side=Right
  t : PMIOPort  Port=4  Side=Left
  w : PMIOPort  Port=5  Side=Right
  t_out : PMIOPort  Port=6  Side=Right
  connections:
  Rigid Transform6/LConn1 -- Rigid Transform5/RConn1
  Rigid Transform16/LConn1 -- Rigid Transform6/RConn1
  Revolute Joint1/LConn1 -- Frame1/RConn1
  Revolute Joint1/RConn3 -- w/RConn1
  Revolute Joint1/LConn2 -- t/RConn1
  Revolute Joint1/RConn2 -- q/RConn1
  Rigid Transform5/LConn1 -- Rigid Transform4/RConn1
  Rigid Transform4/LConn1 -- Revolute Joint1/RConn1
  Solid2/RConn1 -- Frame2/RConn1 -- Reference Frame1/RConn1 -- Rigid Transform16/RConn1
  Revolute Joint1/RConn4 -- t_out/RConn1

== system animation/Plant/Link3 ==
  Reference Frame2 : sm_lib/Frames and Transforms/Reference Frame
  Revolute Joint2 : sm_lib/Joints/Revolute Joint  SenseConstraintForce=off  SenseConstraintForceX=off  SenseConstraintForceY=off  SenseConstraintForceZ=off  SenseConstraintTorque=off  SenseConstraintTorqueX=off  SenseConstraintTorqueY=off  SenseConstraintTorqueZ=off  SenseTotalForce=off  SenseTotalForceX=off  SenseTotalForceY=off  SenseTotalForceZ=off  SenseTotalTorque=off  SenseTotalTorqueX=off  SenseTotalTorqueY=off  SenseTotalTorqueZ=off  CompositeWrenchDir=FollowerOnBase  CompositeWrenchFrame=BaseFrame  EquilibriumPosition=0  EquilibriumPositionUnits=deg  SpringStiffness=0  SpringStiffnessUnits=N*m/deg  DampingCoefficient=0  DampingCoefficientUnits=N*m/(deg/s)  TorqueActuationMode=InputTorque  MotionActuationMode=ComputedMotion  SensePosition=on  SenseVelocity=on  SenseAcceleration=off  SenseTorqueForce=on  PositionTargetSpecify=on  PositionTargetPriority=High  PositionTargetValue=0  PositionTargetValueUnits=deg  VelocityTargetSpecify=on  VelocityTargetPriority=High  VelocityTargetValue=0  VelocityTargetValueUnits=deg/s
  Rigid Transform18 : sm_lib/Frames and Transforms/Rigid Transform  TranslationMethod=None  TranslationStandardOffset=500  TranslationLengthUnit=mm  TranslationStandardAxis=+X  TranslationCartesianOffset=[0 0 0]  TranslationROffset=0  TranslationROffsetUnits=m  TranslationZOffset=0  TranslationZOffsetUnits=m  TranslationThetaOffset=0  TranslationThetaOffsetUnits=deg  RotationMethod=StandardAxis  RotationAngleUnits=rad  RotationStandardAxis=+X  RotationAngle=-pi/2  RotationArbitraryAxis=[0 0 1]  FollAlignAxisA=+X  BaseAlignAxisA=+Y  FollAlignAxisB=+Y  BaseAlignAxisB=+Z  RotationSequenceAxes=FollowerAxes  RotationSequence=XYX  RotationSequenceAngles=[0 0 0]  RotationSequenceAnglesUnits=deg  RotationMatrix=[1 0 0; 0 1 0; 0 0 1]
  Rigid Transform7 : sm_lib/Frames and Transforms/Rigid Transform  TranslationMethod=None  TranslationStandardOffset=0  TranslationLengthUnit=m  TranslationStandardAxis=+Z  TranslationCartesianOffset=[0 0 0]  TranslationROffset=0  TranslationROffsetUnits=m  TranslationZOffset=0  TranslationZOffsetUnits=m  TranslationThetaOffset=0  TranslationThetaOffsetUnits=deg  RotationMethod=StandardAxis  RotationAngleUnits=rad  RotationStandardAxis=+Z  RotationAngle=-pi/3  RotationArbitraryAxis=[0 0 1]  FollAlignAxisA=+X  BaseAlignAxisA=+Y  FollAlignAxisB=+Y  BaseAlignAxisB=+Z  RotationSequenceAxes=FollowerAxes  RotationSequence=XYX  RotationSequenceAngles=[0 0 0]  RotationSequenceAnglesUnits=deg  RotationMatrix=[1 0 0; 0 1 0; 0 0 1]
  Rigid Transform8 : sm_lib/Frames and Transforms/Rigid Transform  TranslationMethod=None  TranslationStandardOffset=250.5  TranslationLengthUnit=mm  TranslationStandardAxis=+Z  TranslationCartesianOffset=[0 0 0]  TranslationROffset=0  TranslationROffsetUnits=m  TranslationZOffset=0  TranslationZOffsetUnits=m  TranslationThetaOffset=0  TranslationThetaOffsetUnits=deg  RotationMethod=None  RotationAngleUnits=deg  RotationStandardAxis=+Z  RotationAngle=0.0  RotationArbitraryAxis=[0 0 1]  FollAlignAxisA=+X  BaseAlignAxisA=+Y  FollAlignAxisB=+Y  BaseAlignAxisB=+Z  RotationSequenceAxes=FollowerAxes  RotationSequence=XYX  RotationSequenceAngles=[0 0 0]  RotationSequenceAnglesUnits=deg  RotationMatrix=[1 0 0; 0 1 0; 0 0 1]
  Rigid Transform9 : sm_lib/Frames and Transforms/Rigid Transform  TranslationMethod=StandardAxis  TranslationStandardOffset=100  TranslationLengthUnit=mm  TranslationStandardAxis=+X  TranslationCartesianOffset=[0 0 0]  TranslationROffset=0  TranslationROffsetUnits=m  TranslationZOffset=0  TranslationZOffsetUnits=m  TranslationThetaOffset=0  TranslationThetaOffsetUnits=deg  RotationMethod=None  RotationAngleUnits=rad  RotationStandardAxis=+X  RotationAngle=pi/2  RotationArbitraryAxis=[0 0 1]  FollAlignAxisA=+X  BaseAlignAxisA=+Y  FollAlignAxisB=+Y  BaseAlignAxisB=+Z  RotationSequenceAxes=FollowerAxes  RotationSequence=XYX  RotationSequenceAngles=[0 0 0]  RotationSequenceAnglesUnits=deg  RotationMatrix=[1 0 0; 0 1 0; 0 0 1]
  Solid3 : sm_lib/Body Elements/Solid  InertiaType=Custom  Mass=1.85  MassUnits=kg  CenterOfMass=[-9.91 0.01 33.80]  CenterOfMassUnits=mm  MomentsOfInertia=[0.02 0.02 0.01]  MomentsOfInertiaUnits=kg*m^2  ProductsOfInertia=[0 0 0]  ProductsOfInertiaUnits=kg*m^2  BasedOnType=Density  Density=1000  DensityUnits=kg/m^3  DoExposeReferenceFrame=on  SerializedFrames=<Frames/>  GraphicType=FromGeometry  MarkerShape=Sphere  MarkerSize=10  GraphicVisPropType=SimpleVisualProperties  GraphicDiffuseColor=[0.0 1.0 1.0]  GraphicSpecularColor=[0.5 0.5 0.5 1.0]  GraphicAmbientColor=[0.15 0.15 0.15 1.0]  GraphicEmissiveColor=[0.0 0.0 0.0 1.0]  GraphicShininess=75  GraphicOpacity=1.0  GeometryShape=FromFile  RectangleSize=[1 1]  RectangleSizeUnits=m  BrickDimensions=[1 1 1]  BrickDimensionUnits=m  CylinderRadius=1  CylinderRadiusUnits=m  CylinderLength=1  CylinderLengthUnits=m  SphereRadius=1  SphereRadiusUnits=m  EllipsoidRadii=[1 1 1]  EllipsoidRadiiUnits=m  ExtrusionCrossSection=[1 1; -1 1; -1 -1; 1 -1]  ExtrusionCrossSectionUnits=m  ExtrusionLength=1  ExtrusionLengthUnits=m  PolygonNumSides=3  PolygonOuterRadius=1  PolygonOuterRadiusUnits=m  ExtGeomFileType=STL  ExtGeomFileName=D:\Chin\3rdYearsProject\IntroRobotics\Project\CAD\SubAssem4.STL  ExtGeomFileUnits=mm  RevolutionCrossSection=[1 1; 1 -1; 2 -1; 2 1]  RevolutionCrossSectionUnits=m  RevolutionExtent=Full  RevolutionAngle=180  RevolutionAngleUnits=deg
  Frame2 : PMIOPort  Side=Left
  t : PMIOPort  Port=2  Side=Left
  Frame3 : PMIOPort  Port=3  Side=Right
  q : PMIOPort  Port=4  Side=Right
  w : PMIOPort  Port=5  Side=Right
  t_out : PMIOPort  Port=6  Side=Right
  connections:
  Solid3/RConn1 -- Frame3/RConn1 -- Rigid Transform18/RConn1 -- Reference Frame2/RConn1
  Rigid Transform7/LConn1 -- Revolute Joint2/RConn1
  Rigid Transform8/LConn1 -- Rigid Transform7/RConn1
  Rigid Transform9/LConn1 -- Rigid Transform8/RConn1
  Rigid Transform9/RConn1 -- Rigid Transform18/LConn1
  Revolute Joint2/LConn1 -- Frame2/RConn1
  Revolute Joint2/RConn3 -- w/RConn1
  Revolute Joint2/LConn2 -- t/RConn1
  Revolute Joint2/RConn2 -- q/RConn1
  t_out/RConn1 -- Revolute Joint2/RConn4

== system animation/Plant/Link4 ==
  Reference Frame3 : sm_lib/Frames and Transforms/Reference Frame
  Revolute Joint3 : sm_lib/Joints/Revolute Joint  SenseConstraintForce=off  SenseConstraintForceX=off  SenseConstraintForceY=off  SenseConstraintForceZ=off  SenseConstraintTorque=off  SenseConstraintTorqueX=off  SenseConstraintTorqueY=off  SenseConstraintTorqueZ=off  SenseTotalForce=off  SenseTotalForceX=off  SenseTotalForceY=off  SenseTotalForceZ=off  SenseTotalTorque=off  SenseTotalTorqueX=off  SenseTotalTorqueY=off  SenseTotalTorqueZ=off  CompositeWrenchDir=FollowerOnBase  CompositeWrenchFrame=BaseFrame  EquilibriumPosition=0  EquilibriumPositionUnits=deg  SpringStiffness=0  SpringStiffnessUnits=N*m/deg  DampingCoefficient=0  DampingCoefficientUnits=N*m/(deg/s)  TorqueActuationMode=InputTorque  MotionActuationMode=ComputedMotion  SensePosition=on  SenseVelocity=on  SenseAcceleration=off  SenseTorqueForce=on  PositionTargetSpecify=on  PositionTargetPriority=High  PositionTargetValue=0  PositionTargetValueUnits=deg  VelocityTargetSpecify=on  VelocityTargetPriority=High  VelocityTargetValue=0  VelocityTargetValueUnits=deg/s
  Rigid Transform10 : sm_lib/Frames and Transforms/Rigid Transform  TranslationMethod=None  TranslationStandardOffset=0  TranslationLengthUnit=m  TranslationStandardAxis=+Z  TranslationCartesianOffset=[0 0 0]  TranslationROffset=0  TranslationROffsetUnits=m  TranslationZOffset=0  TranslationZOffsetUnits=m  TranslationThetaOffset=0  TranslationThetaOffsetUnits=deg  RotationMethod=None  RotationAngleUnits=rad  RotationStandardAxis=+Z  RotationAngle=-pi/2  RotationArbitraryAxis=[0 0 1]  FollAlignAxisA=+X  BaseAlignAxisA=+Y  FollAlignAxisB=+Y  BaseAlignAxisB=+Z  RotationSequenceAxes=FollowerAxes  RotationSequence=XYX  RotationSequenceAngles=[0 0 0]  RotationSequenceAnglesUnits=deg  RotationMatrix=[1 0 0; 0 1 0; 0 0 1]
  Rigid Transform11 : sm_lib/Frames and Transforms/Rigid Transform  TranslationMethod=StandardAxis  TranslationStandardOffset=507.2  TranslationLengthUnit=mm  TranslationStandardAxis=-Z  TranslationCartesianOffset=[0 0 0]  TranslationROffset=0  TranslationROffsetUnits=m  TranslationZOffset=0  TranslationZOffsetUnits=m  TranslationThetaOffset=0  TranslationThetaOffsetUnits=deg  RotationMethod=None  RotationAngleUnits=deg  RotationStandardAxis=+Z  RotationAngle=0.0  RotationArbitraryAxis=[0 0 1]  FollAlignAxisA=+X  BaseAlignAxisA=+Y  FollAlignAxisB=+Y  BaseAlignAxisB=+Z  RotationSequenceAxes=FollowerAxes  RotationSequence=XYX  RotationSequenceAngles=[0 0 0]  RotationSequenceAnglesUnits=deg  RotationMatrix=[1 0 0; 0 1 0; 0 0 1]
  Rigid Transform12 : sm_lib/Frames and Transforms/Rigid Transform  TranslationMethod=None  TranslationStandardOffset=0  TranslationLengthUnit=m  TranslationStandardAxis=+Z  TranslationCartesianOffset=[0 0 0]  TranslationROffset=0  TranslationROffsetUnits=m  TranslationZOffset=0  TranslationZOffsetUnits=m  TranslationThetaOffset=0  TranslationThetaOffsetUnits=deg  RotationMethod=None  RotationAngleUnits=rad  RotationStandardAxis=+X  RotationAngle=pi/2  RotationArbitraryAxis=[0 0 1]  FollAlignAxisA=+X  BaseAlignAxisA=+Y  FollAlignAxisB=+Y  BaseAlignAxisB=+Z  RotationSequenceAxes=FollowerAxes  RotationSequence=XYX  RotationSequenceAngles=[0 0 0]  RotationSequenceAnglesUnits=deg  RotationMatrix=[1 0 0; 0 1 0; 0 0 1]
  Rigid Transform19 : sm_lib/Frames and Transforms/Rigid Transform  TranslationMethod=None  TranslationStandardOffset=500  TranslationLengthUnit=mm  TranslationStandardAxis=+X  TranslationCartesianOffset=[0 0 0]  TranslationROffset=0  TranslationROffsetUnits=m  TranslationZOffset=0  TranslationZOffsetUnits=m  TranslationThetaOffset=0  TranslationThetaOffsetUnits=deg  RotationMethod=StandardAxis  RotationAngleUnits=rad  RotationStandardAxis=+X  RotationAngle=pi/2  RotationArbitraryAxis=[0 0 1]  FollAlignAxisA=+X  BaseAlignAxisA=+Y  FollAlignAxisB=+Y  BaseAlignAxisB=+Z  RotationSequenceAxes=FollowerAxes  RotationSequence=XYX  RotationSequenceAngles=[0 0 0]  RotationSequenceAnglesUnits=deg  RotationMatrix=[1 0 0; 0 1 0; 0 0 1]
  Solid4 : sm_lib/Body Elements/Solid  InertiaType=Custom  Mass=1.735  MassUnits=kg  CenterOfMass=[0.09 234.59 -19.21]  CenterOfMassUnits=mm  MomentsOfInertia=[0.13 0.01 0.13]  MomentsOfInertiaUnits=kg*m^2  ProductsOfInertia=[-0.01 0 0]  ProductsOfInertiaUnits=kg*m^2  BasedOnType=Density  Density=1000  DensityUnits=kg/m^3  DoExposeReferenceFrame=on  SerializedFrames=<Frames/>  GraphicType=FromGeometry  MarkerShape=Sphere  MarkerSize=10  GraphicVisPropType=SimpleVisualProperties  GraphicDiffuseColor=[1.0 0.2 0.2]  GraphicSpecularColor=[0.5 0.5 0.5 1.0]  GraphicAmbientColor=[0.15 0.15 0.15 1.0]  GraphicEmissiveColor=[0.0 0.0 0.0 1.0]  GraphicShininess=75  GraphicOpacity=1.0  GeometryShape=FromFile  RectangleSize=[1 1]  RectangleSizeUnits=m  BrickDimensions=[1 1 1]  BrickDimensionUnits=m  CylinderRadius=1  CylinderRadiusUnits=m  CylinderLength=1  CylinderLengthUnits=m  SphereRadius=1  SphereRadiusUnits=m  EllipsoidRadii=[1 1 1]  EllipsoidRadiiUnits=m  ExtrusionCrossSection=[1 1; -1 1; -1 -1; 1 -1]  ExtrusionCrossSectionUnits=m  ExtrusionLength=1  ExtrusionLengthUnits=m  PolygonNumSides=3  PolygonOuterRadius=1  PolygonOuterRadiusUnits=m  ExtGeomFileType=STL  ExtGeomFileName=D:\Chin\3rdYearsProject\IntroRobotics\Project\CAD\SubAssem5.STL  ExtGeomFileUnits=mm  RevolutionCrossSection=[1 1; 1 -1; 2 -1; 2 1]  RevolutionCrossSectionUnits=m  RevolutionExtent=Full  RevolutionAngle=180  RevolutionAngleUnits=deg
  Frame4 : PMIOPort  Side=Left
  Frame3 : PMIOPort  Port=2  Side=Right
  t : PMIOPort  Port=3  Side=Left
  q : PMIOPort  Port=4  Side=Right
  w : PMIOPort  Port=5  Side=Right
  t_out : PMIOPort  Port=6  Side=Right
  connections:
  Revolute Joint3/RConn3 -- w/RConn1
  Revolute Joint3/RConn2 -- q/RConn1
  Revolute Joint3/LConn2 -- t/RConn1
  Rigid Transform11/LConn1 -- Rigid Transform10/RConn1
  Rigid Transform12/LConn1 -- Rigid Transform11/RConn1
  Solid4/RConn1 -- Frame4/RConn1 -- Rigid Transform19/RConn1 -- Reference Frame3/RConn1
  Rigid Transform10/LConn1 -- Revolute Joint3/RConn1
  Rigid Transform12/RConn1 -- Rigid Transform19/LConn1
  Revolute Joint3/LConn1 -- Frame3/RConn1
  t_out/RConn1 -- Revolute Joint3/RConn4
